simulink model "envelope_simulink"  (R2017a)
settings: Solver=VariableStepAuto  StartTime=0.0  StopTime=10.0  RelTol=1e-3
undefined symbols (not defined in the file or in its folder): DiscIntNeverNeededParam
settings Model: Creator=Andre  LastModifiedBy=Andre

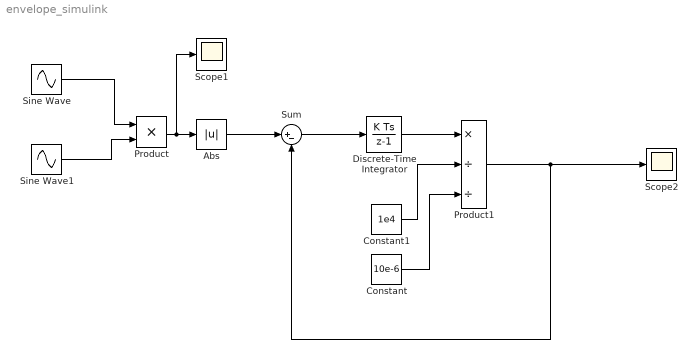
== system envelope_simulink ==
  Abs : Abs
  Constant : Constant  Value=10e-6
  Constant1 : Constant  Value=1e4
  Discrete-Time Integrator : DiscreteIntegrator  InitialConditionSetting=State (most efficient)  SampleTime=-1  ICPrevOutput=DiscIntNeverNeededParam  ICPrevScaledInput=DiscIntNeverNeededParam
  Product : Product
  Product1 : Product  Inputs=*//
  Scope1 : Scope
  Scope2 : Scope
  Sine Wave : Sin  Frequency=100  SampleTime=0
  Sine Wave1 : Sin  SampleTime=0
  Sum : Sum  Inputs=|+-
  wires:
  Sine Wave/1 -> Product/1
  Sine Wave1/1 -> Product/2
  Product/1 -> Scope1/1, Abs/1
  Constant/1 -> Product1/3
  Constant1/1 -> Product1/2
  Discrete-Time Integrator/1 -> Product1/1
  Abs/1 -> Sum/1
  Product1/1 -> Scope2/1, Sum/2
  Sum/1 -> Discrete-Time Integrator/1
